simulink model "Q2_SP_Full_Wave_Rectifier"  (R2018a)
settings: Solver=VariableStepAuto  StartTime=0.0  StopTime=10  FixedStep=10e-06  MaxStep=1e-5  MinStep=1e-7  RelTol=1e-3
libraries: powerlib x15, powerlib_meascontrol x2, pePowerMeasurement x2
settings Model: SimulationMode=accelerator  Creator=Emre Deniz  LastModifiedBy=Furkan

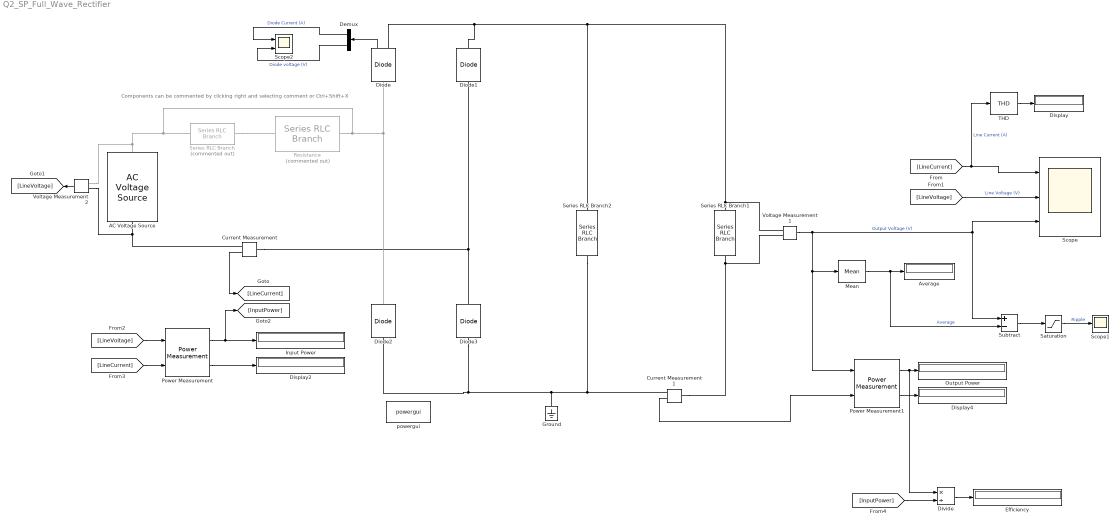
== system Q2_SP_Full_Wave_Rectifier ==
  note: Components can be commented by clicking right and selecting comment or Ctrl+Shift+X
  AC Voltage Source : powerlib/Electrical Sources/AC Voltage Source  Amplitude=230 * sqrt(2)  Phase=0  Frequency=50  SampleTime=0  Measurements=None  BusType=swing  Pref=10e3  Qref=0  Qmin=-inf  Qmax=+inf
  Average : Display
  Current Measurement : powerlib/Measurements/Current Measurement  PhasorSimulation=off  OutputType=Complex  PSBequivalent=0
  Current Measurement1 : powerlib/Measurements/Current Measurement  PhasorSimulation=off  OutputType=Complex  PSBequivalent=0
  Demux : Demux  Outputs=2
  Diode : powerlib/Power Electronics/Diode  Ron=1e-3  Lon=0  Vf=0  IC=0  UseSnubber=0  Rs=0  Cs=0  Measurements=on
  Diode1 : powerlib/Power Electronics/Diode  Ron=1e-3  Lon=0  Vf=0  IC=0  UseSnubber=0  Rs=0  Cs=0  Measurements=off
  Diode2 : powerlib/Power Electronics/Diode  Ron=0  Lon=0  Vf=0  IC=0  UseSnubber=0  Rs=0  Cs=0  Measurements=off
  Diode3 : powerlib/Power Electronics/Diode  Ron=0  Lon=0  Vf=0  IC=0  UseSnubber=0  Rs=0  Cs=0  Measurements=off
  Display : Display
      settings: Decimation=4
  Display2 : Display
  Display4 : Display
  Divide : Product  Inputs=*/
  Efficiency : Display
  Ground : powerlib/Elements/Ground  LConnTagsString=a
  Input Power : Display
  Mean : powerlib_meascontrol/Measurements/Mean  Freq=50  Vinit=0  Ts=0
  Output Power : Display
  Power Measurement : pePowerMeasurement/Power Measurement  OverrideUsingVariant=Continuous  F=50  K=[1]  Ts=0
  Power Measurement1 : pePowerMeasurement/Power Measurement  OverrideUsingVariant=Continuous  F=50  K=[0]  Ts=0
  Resistance : powerlib/Elements/Series RLC Branch  Commented=on  LConnTagsString=__new0  RConnTagsString=__new0  BranchType=R  Resistance=0.8e-03  Inductance=0  SetiL0=off  InitialCurrent=0  Capacitance=0  Setx0=off  InitialVoltage=0  Measurements=None
  Saturation : Saturate  UpperLimit=+5  LowerLimit=-5
  Scope : Scope  NumInputPorts=3
  Scope1 : Scope
  Scope2 : Scope  NumInputPorts=2
  Series RLC Branch : powerlib/Elements/Series RLC Branch  Commented=on  LConnTagsString=__new0  RConnTagsString=__new0  BranchType=L  Resistance=1  Inductance=1.3e-03  SetiL0=off  InitialCurrent=0  Capacitance=1e-6  Setx0=off  InitialVoltage=0  Measurements=None
  Series RLC Branch1 : powerlib/Elements/Series RLC Branch  LConnTagsString=__new0  RConnTagsString=__new0  BranchType=R  Resistance=70  Inductance=1e-3  SetiL0=off  InitialCurrent=0  Capacitance=1e-6  Setx0=off  InitialVoltage=0  Measurements=Branch voltage
  Series RLC Branch2 : powerlib/Elements/Series RLC Branch  LConnTagsString=__new0  RConnTagsString=__new0  BranchType=C  Resistance=1  Inductance=1e-3  SetiL0=off  InitialCurrent=0  Capacitance=8.2e-3  Setx0=on  InitialVoltage=300  Measurements=None
  Subtract : Sum  Inputs=+-
  THD : powerlib_meascontrol/Measurements/THD  Freq=50  Ts=0
  Voltage Measurement1 : powerlib/Measurements/Voltage Measurement  PhasorSimulation=off  OutputType=Complex  PSBequivalent=0
  Voltage Measurement2 : powerlib/Measurements/Voltage Measurement  PhasorSimulation=off  OutputType=Complex  PSBequivalent=0
  powergui : powerlib/powergui  Priority=1  SimulationMode=Continuous  SampleTime=10e-6  frequency=60  Iterations=50  frequencyindice=50  Pbase=100e6  ErrMax=1e-4  UnitsV=kV  UnitsW=MW  buscounter=0  FunctionMessages=off  echomessages=off  EnableUseOfTLC=off  CurrentSourceSwitches=off  DisableSnubberDevices=off  DisableRonSwitches=off  DisableVfSwitches=off  DisplayEquations=off  SolverType=Tustin/Backward Euler (TBE)  Interpol=off  ExternalGateDelay=off  methode=off  Ts=100  x0status=blocks  SPID=off  SwTol=0  HookPort=off  RestoreLinks=warning  ResistiveCurrentMeasurement=off  Frange=[0:2:500]  Ylog=off  Xlog=on  ShowGrid=off  save=off  variable=ZData  structure=0  ZoomFFT=off  StartTime=0.0  cycles=1  DisplayStyle=1  fundamental=60  FreqAxis=off  MaxFrequency=1000  frequencyindicesteady=1  RmsSteady=1  display=off
  wires:
  Voltage Measurement1/1 -> Power Measurement1/1, Mean/1, Subtract/1, Scope/3  "Output Voltage (V)"
  Mean/1 -> Subtract/2, Average/1  "Average"
  Subtract/1 -> Saturation/1
  Saturation/1 -> Scope1/1  "Ripple"
  Current Measurement/1 -> [LineCurrent]
  Voltage Measurement2/1 -> [LineVoltage]
  [LineVoltage] -> Scope/2  "Line Voltage (V)"
  [LineCurrent] -> THD/1, Scope/1  "Line Current (A)"
  THD/1 -> Display/1
  Diode/1 -> Demux/1
  Demux/1 -> Scope2/1  "Diode Current (A)"
  Demux/2 -> Scope2/2  "Diode voltage (V)"
  [LineVoltage] -> Power Measurement/1
  [LineCurrent] -> Power Measurement/2
  Power Measurement/1 -> [InputPower], Input Power/1
  Power Measurement/2 -> Display2/1
  Current Measurement1/1 -> Power Measurement1/2
  Power Measurement1/1 -> Divide/1, Output Power/1
  Power Measurement1/2 -> Display4/1
  [InputPower] -> Divide/2
  Divide/1 -> Efficiency/1
  connections:
  Series RLC Branch/RConn1 -- Resistance/LConn1
  Series RLC Branch1/RConn1 -- Current Measurement1/LConn1 -- Voltage Measurement1/LConn2
  Diode3/RConn1 -- Current Measurement/LConn1 -- Diode1/LConn1
  Diode/RConn1 -- Voltage Measurement1/LConn1 -- Series RLC Branch1/LConn1 -- Series RLC Branch2/LConn1 -- Diode1/RConn1
  Current Measurement/RConn1 -- Voltage Measurement2/LConn2 -- AC Voltage Source/LConn1
  Series RLC Branch/LConn1 -- Diode2/RConn1 -- Diode/LConn1 -- Resistance/RConn1 -- Voltage Measurement2/LConn1 -- AC Voltage Source/RConn1
  Diode3/LConn1 -- Ground/LConn1 -- Current Measurement1/RConn1 -- Series RLC Branch2/RConn1 -- Diode2/LConn1
